simulink model "Lights"  (Simulink 6.4)
settings: Solver=ode45  StartTime=0.0  StopTime=5000  RelTol=1e-3
libraries: simulink x5, Sensors_Lib x1
settings Model: Creator=VMAdmin  LastModifiedBy=VMAdmin
settings DataIOCC: SaveFormat=Structure
settings DebuggingCC: SignalResolutionControl=UseLocalSettings  MultiTaskDSMMsg=error  MultiTaskCondExecSysMsg=error
settings GRTTargetCC: TargetFcnLib=ansi_tfl_table_tmw.mat

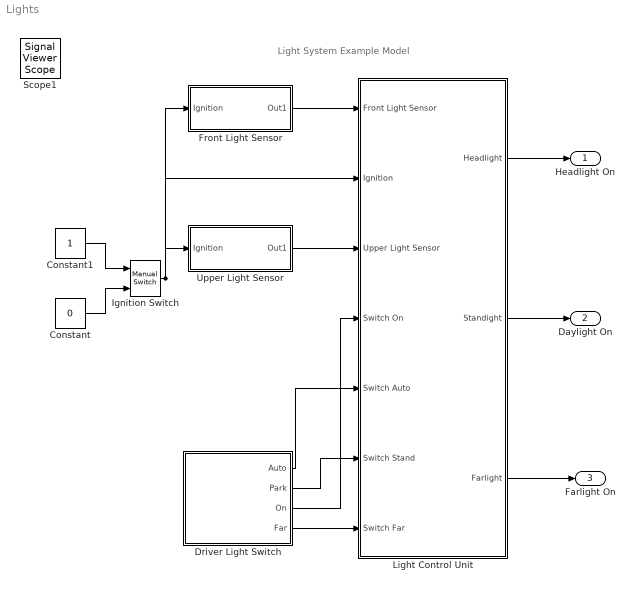
== system Lights ==
  note: Light System Example Model
  Constant : Constant  Value=0  OutDataType=sfix(16)  ConRadixGroup=Use specified scaling  OutScaling=2^0  SampleTime=inf  FramePeriod=inf
  Constant1 : Constant  Value=1  OutDataType=sfix(16)  ConRadixGroup=Use specified scaling  OutScaling=2^0  SampleTime=inf  FramePeriod=inf
  Driver Light Switch : Subsystem
  Front Light Sensor : Subsystem  AncestorBlock=Sensors_Lib/Front Light Sensor
  Ignition Switch : simulink/Signal Routing/Manual Switch  SystemSampleTime=-1  sw=0  action=0
  Light Control Unit : Subsystem  mask{do_init=off}
      mask prompts: do_init "activate initial setting"
      mask help:
      | masked subsystem
      | demonstration mode
  Upper Light Sensor : Subsystem  AncestorBlock=Sensors_Lib/Upper Light Sensor
  Headlight On : Outport
  Daylight On : Outport  Port=2
  Farlight On : Outport  Port=3
  Scope1 : SignalViewerScope  IOType=viewer  RefreshTime=0.035000
  wires:
  Ignition Switch/1 -> Light Control Unit/2(Ignition), Front Light Sensor/1(Ignition), Upper Light Sensor/1(Ignition)
  Driver Light Switch/1(Auto) -> Light Control Unit/5(Switch Auto)
  Driver Light Switch/2(Park) -> Light Control Unit/6(Switch Stand)
  Driver Light Switch/3(On) -> Light Control Unit/4(Switch On)
  Driver Light Switch/4(Far) -> Light Control Unit/7("Switch Far ")
  Constant1/1 -> Ignition Switch/1
  Constant/1 -> Ignition Switch/2
  Front Light Sensor/1(Out1) -> Light Control Unit/1(Front Light Sensor)
  Upper Light Sensor/1(Out1) -> Light Control Unit/3(Upper Light Sensor)
  Light Control Unit/1(Headlight) -> Headlight On/1
  Light Control Unit/2(Standight) -> Daylight On/1
  Light Control Unit/3(Farlight) -> Farlight On/1

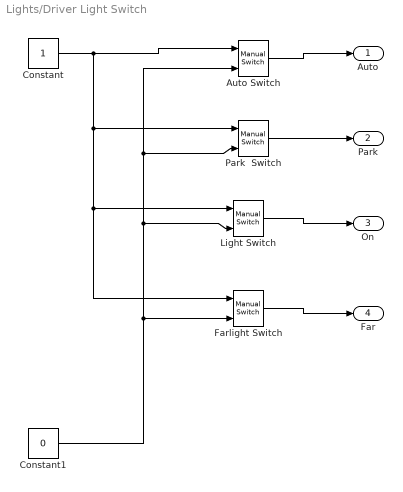
== system Lights/Driver Light Switch ==
  Auto Switch : simulink/Signal Routing/Manual Switch  SystemSampleTime=-1  sw=1  action=0  varsize=off
  Constant : Constant  Value=1  OutDataTypeMode=boolean  OutDataType=sfix(16)  ConRadixGroup=Use specified scaling  OutScaling=2^0  SampleTime=inf  FramePeriod=inf
  Constant1 : Constant  Value=0  OutDataTypeMode=boolean  OutDataType=sfix(16)  ConRadixGroup=Use specified scaling  OutScaling=2^0  SampleTime=inf  FramePeriod=inf
  Farlight Switch : simulink/Signal Routing/Manual Switch  SystemSampleTime=-1  sw=1  action=0  varsize=off
  Light Switch : simulink/Signal Routing/Manual Switch  SystemSampleTime=-1  sw=0  action=0  varsize=off
  Park  Switch : simulink/Signal Routing/Manual Switch  SystemSampleTime=-1  sw=0  action=0  varsize=off
  Auto : Outport  DataType=boolean
  Park : Outport  Port=2
  On : Outport  Port=3
  Far : Outport  Port=4
  wires:
  Constant1/1 -> Auto Switch/2, Park  Switch/2, Light Switch/2, Farlight Switch/2
  Auto Switch/1 -> Auto/1
  Constant/1 -> Auto Switch/1, Park  Switch/1, Light Switch/1, Farlight Switch/1
  Park  Switch/1 -> Park/1
  Light Switch/1 -> On/1
  Farlight Switch/1 -> Far/1

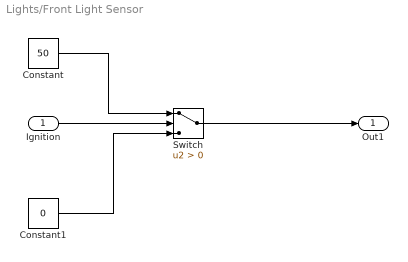
== system Lights/Front Light Sensor ==
  Ignition : Inport
  Constant : Constant  Value=50  OutDataType=sfix(16)  ConRadixGroup=Use specified scaling  OutScaling=2^0  SampleTime=inf  FramePeriod=inf
  Constant1 : Constant  Value=0  OutDataType=sfix(16)  ConRadixGroup=Use specified scaling  OutScaling=2^0  SampleTime=inf  FramePeriod=inf
  Switch : Switch  Criteria=u2 > Threshold
  Out1 : Outport
  wires:
  Switch/1 -> Out1/1
  Constant1/1 -> Switch/3
  Ignition/1 -> Switch/2
  Constant/1 -> Switch/1

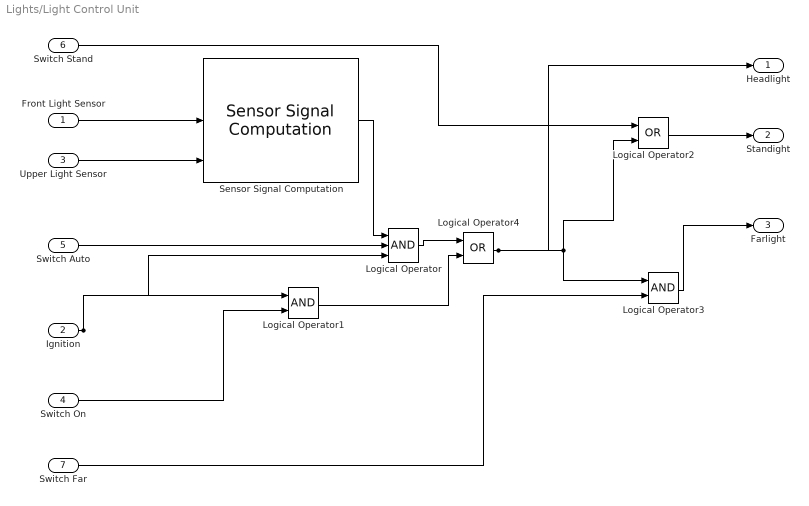
== system Lights/Light Control Unit ==
  Front Light Sensor : Inport
  Ignition : Inport  Port=2
  Upper Light Sensor : Inport  Port=3
  Switch On : Inport  Port=4
  Switch Auto : Inport  Port=5
  Switch Stand : Inport  Port=6
  "Switch Far " : Inport  Port=7
  Logical Operator : Logic  Inputs=3  AllPortsSameDT=off  OutDataTypeMode=Boolean
  Logical Operator1 : Logic  AllPortsSameDT=off  OutDataTypeMode=Boolean
  Logical Operator2 : Logic  Operator=OR  AllPortsSameDT=off  OutDataTypeMode=Boolean
  Logical Operator3 : Logic  AllPortsSameDT=off  OutDataTypeMode=Boolean
  Logical Operator4 : Logic  Operator=OR  AllPortsSameDT=off  OutDataTypeMode=Boolean
  "Sensor Signal Computation " : Sensors_Lib/Sensor Signal Computation   SystemSampleTime=-1
  Headlight : Outport
  Standight : Outport  Port=2
  Farlight : Outport  Port=3
  wires:
  Ignition/1 -> Logical Operator/3, Logical Operator1/1
  Logical Operator3/1 -> Farlight/1
  Logical Operator2/1 -> Standight/1
  Switch Stand/1 -> Logical Operator2/1
  Switch On/1 -> Logical Operator1/2
  Logical Operator/1 -> Logical Operator4/1
  Logical Operator1/1 -> Logical Operator4/2
  Logical Operator4/1 -> Headlight/1, Logical Operator2/2, Logical Operator3/1
  "Switch Far "/1 -> Logical Operator3/2
  Front Light Sensor/1 -> "Sensor Signal Computation "/2
  Upper Light Sensor/1 -> "Sensor Signal Computation "/3
  Switch Auto/1 -> Logical Operator/2
  "Sensor Signal Computation "/1 -> Logical Operator/1

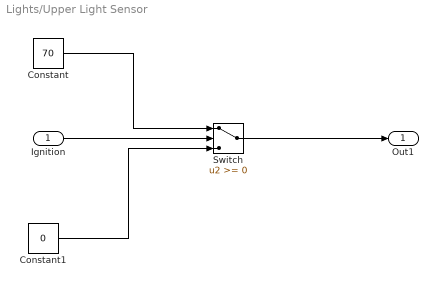
== system Lights/Upper Light Sensor ==
  Ignition : Inport
  Constant : Constant  Value=70  OutDataType=sfix(16)  ConRadixGroup=Use specified scaling  OutScaling=2^0  SampleTime=inf  FramePeriod=inf
  Constant1 : Constant  Value=0  OutDataType=sfix(16)  ConRadixGroup=Use specified scaling  OutScaling=2^0  SampleTime=inf  FramePeriod=inf
  Switch : Switch
  Out1 : Outport
  wires:
  Ignition/1 -> Switch/2
  Constant/1 -> Switch/1
  Constant1/1 -> Switch/3
  Switch/1 -> Out1/1
